simulink model "DC_core_control"  (R2023b)
settings: configuration reference "ctrl_tsk_conf" (kept outside this file)
undefined symbols (not defined in the file): ctrl_tsk_st, dcBusCtrl, shuntMaxRequestedCurrentrms
libraries: eeGeneralControl x2, simulink x1, slpidlib x1
settings Model: DataDictionary=fmuGenerationDictionay.sldd  Creator=Veimar  LastModifiedBy=Veimar
settings ConfigSetRef: SourceName=ctrl_tsk_conf

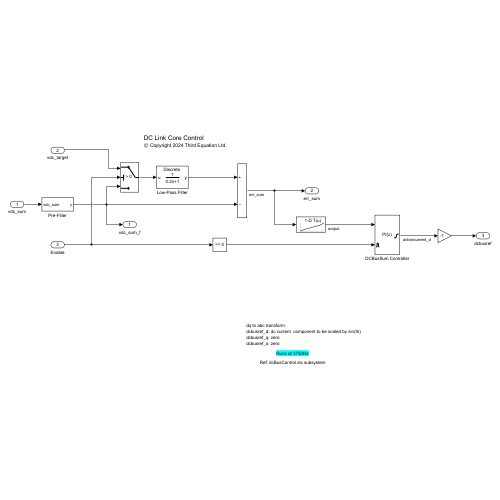
[thumbnail: Simulink's stored preview of the top-level diagram]
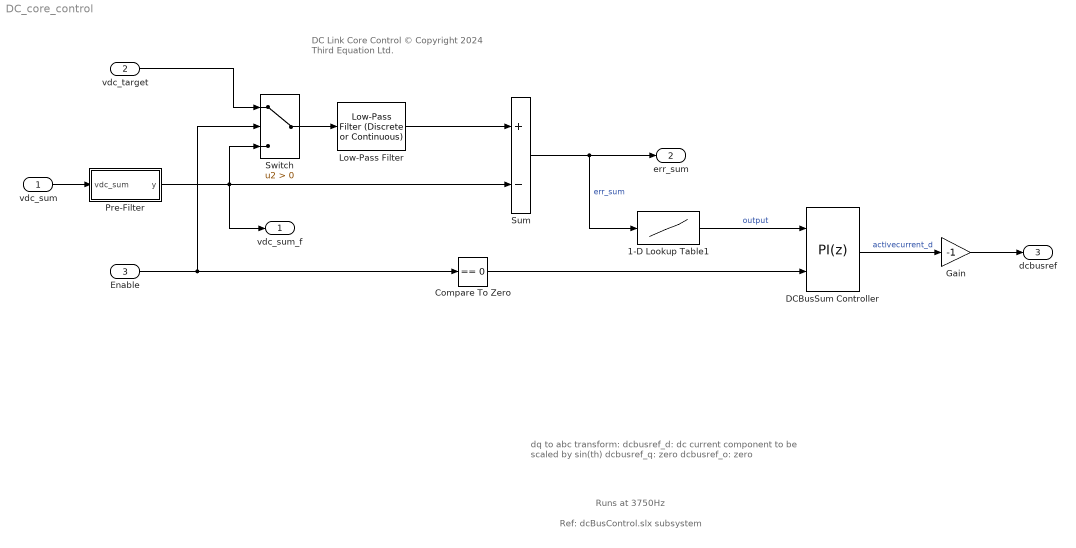
== system DC_core_control ==
  note: Runs at 3750Hz
  note: Ref: dcBusControl.slx subsystem
  note: dq to abc transform:
      | dcbusref_d: dc current  component to be scaled by sin(th)
      | dcbusref_q: zero
      | dcbusref_o: zero
  note: DC Link Core Control
      | © Copyright 2024 Third Equation Ltd.
  vdc_sum : Inport  OutDataTypeStr=single  PortDimensions=1
  vdc_target : Inport  Port=2  OutDataTypeStr=single  PortDimensions=1
  Enable : Inport  Port=3  OutDataTypeStr=boolean  PortDimensions=1
  1-D Lookup Table1 : Lookup_n-D  NumberOfTableDimensions=1  BreakpointsForDimension1=[-15 -10 10 15]  Table=[-20 -10 10 20]  InternalRulePriority=Speed  RndMeth=Simplest
  Compare To Zero : simulink/Logic and Bit Operations/Compare To Zero  relop===  OutDataTypeStr=boolean
  DCBusSum Controller : slpidlib/PID Controller  Controller=PI  Form=Parallel  TimeDomain=Discrete-time  UseExternalTs=off  SampleTime=-1  IntegratorMethod=Forward Euler  FilterMethod=Forward Euler  ControllerParametersSource=internal  P=dcBusCtrl.Sum.PGain  I=dcBusCtrl.Sum.IGain  UseKiTs=off  D=0  N=100  UseFilter=on  TunerSelectOption=Frequency Response Based  InitialConditionSource=internal  InitialConditionForIntegrator=0  InitialConditionForFilter=0  DifferentiatorICPrevScaledInput=0  ExternalReset=level  TrackingMode=off  Kt=1  LimitOutput=on  SatLimitsSource=internal  UpperSaturationLimit=shuntMaxRequestedCurrentrms*sqrt(2)  LowerSaturationLimit=-shuntMaxRequestedCurrentrms*sqrt(2)  LinearizeAsGain=on  AntiWindupMode=clamping  Kb=1  LimitIntegrator=off  UpperIntegratorSaturationLimit=inf  LowerIntegratorSaturationLimit=-inf  POutMin=[]  POutMax=[]  IOutMin=[]  IOutMax=[]  DOutMin=[]  DOutMax=[]  NOutMin=[]  NOutMax=[]  SumOutMin=[]  SumOutMax=[]  SaturationOutMin=[]  SaturationOutMax=[]  PParamMin=[]  PParamMax=[]  IParamMin=[]  IParamMax=[]  DParamMin=[]  DParamMax=[]  NParamMin=[]  NParamMax=[]  KbParamMin=[]  KbParamMax=[]  KtParamMin=[]  KtParamMax=[]  KbOutMin=[]  KbOutMax=[]  KtOutMin=[]  KtOutMax=[]  IntegratorOutMin=[]  IntegratorOutMax=[]  FilterOutMin=[]  FilterOutMax=[]  SumI1OutMin=[]  SumI1OutMax=[]  SumI2OutMin=[]  SumI2OutMax=[]  SumI3OutMin=[]  SumI3OutMax=[]  SumI4OutMin=[]  SumI4OutMax=[]  SumDOutMin=[]  SumDOutMax=[]  DifferentiatorOutMin=[]  DifferentiatorOutMax=[]  FilterDiffOutCoefMin=[]  FilterDiffOutCoefMax=[]  ReciprocalOutMin=[]  ReciprocalOutMax=[]  SumDenOutMin=[]  SumDenOutMax=[]  SumNumOutMin=[]  SumNumOutMax=[]  DivideOutMin=[]  DivideOutMax=[]  UdiffTsProdOutMin=[]  UdiffTsProdOutMax=[]  NTsProdOutMin=[]  NTsProdOutMax=[]  UintegralTsProdOutMin=[]  UintegralTsProdOutMax=[]  UngainTsProdOutMin=[]  UngainTsProdOutMax=[]  ClampingZeroOutDataTypeStr=Inherit: Inherit via back propagation  ClampingZeroOutMin=[]  ClampingZeroOutMax=[]  FilterDenConstantOutDataTypeStr=Inherit: Inherit via back propagation  FilterDenConstantOutMin=[]  FilterDenConstantOutMax=[]  PCopyOutDataTypeStr=Inherit: Inherit via back propagation  PCopyOutMin=[]  PCopyOutMax=[]  NCopyOutDataTypeStr=Inherit: Inherit via back propagation  NCopyOutMin=[]  NCopyOutMax=[]  IntegratorContinuousStateAttributes=''  IntegratorStateMustResolveToSignalObject=off  IntegratorRTWStateStorageClass=Auto  FilterContinuousStateAttributes=''  FilterStateMustResolveToSignalObject=off  FilterRTWStateStorageClass=Auto  ParallelPVariant=InternalParameters  IdealPVariant=Disabled  IVariant=InternalParameters  DVariant=Disabled  IntegratorVariant=Discrete  SatVariant=Enabled  AWVariant=DiscClampingParallel  PCopyVariant=Disabled  TRVariant=Disabled  FdbkBlocksVariant=Forward  IdealPFdbkVariant=Disabled  SatFdbkVariant=Disabled  DerivativeFilterVariant=Disabled  NVariant=Disabled  NCopyVariant=Disabled_SignalSpec  FilterICVariant=Disabled  IntegratorICVariant=InternalICs  ExternalResetVariant=ExternalReset  TRSumVariant=Passthrough  SumFdbkVariant=Disabled  SumVariant=Sum_PI  TsampFilterVariant=InternalTs  TsampNgainVariant=Passthrough  TsampIntegralVariant=Disabled_SignalSpec  ExternalSaturationOutDataTypeStr=Inherit: Same as second input
  Gain : Gain  Gain=-1
  Low-Pass Filter : eeGeneralControl/Low-Pass Filter (Discrete or Continuous)  K=1  T=0.2  B=inf  A=-inf  init_option=Inherited from block input  x0=0  Ts=-1
  Pre-Filter : Subsystem
  Sum : Sum  Inputs=+-
  Switch : Switch  Criteria=u2 > Threshold  SaturateOnIntegerOverflow=off  InputSameDT=off
  vdc_sum_f : Outport  OutDataTypeStr=single  PortDimensions=1
  err_sum : Outport  Port=2  OutDataTypeStr=single  PortDimensions=1
  dcbusref : Outport  Port=3  OutDataTypeStr=single  PortDimensions=1
  wires:
  Enable/1 -> Switch/2, Compare To Zero/1
  Sum/1 -> 1-D Lookup Table1/1, err_sum/1  "err_sum"
  Pre-Filter/1(y) -> vdc_sum_f/1, Sum/2, Switch/3
  1-D Lookup Table1/1 -> DCBusSum Controller/1  "output"
  DCBusSum Controller/1 -> Gain/1  "activecurrent_d"
  vdc_sum/1 -> Pre-Filter/1(vdc_sum)
  Gain/1 -> dcbusref/1
  Switch/1 -> Low-Pass Filter/1
  vdc_target/1 -> Switch/1
  Low-Pass Filter/1 -> Sum/1
  Compare To Zero/1 -> DCBusSum Controller/2

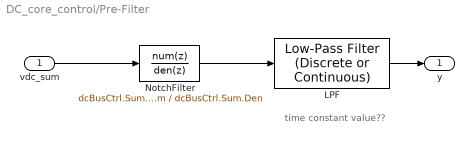
== system DC_core_control/Pre-Filter ==
  note: time constant value??
  vdc_sum : Inport
  LPF : eeGeneralControl/Low-Pass Filter (Discrete or Continuous)  K=1  T=1/(100 * 2 * pi)  B=inf  A=-inf  init_option=Inherited from block input  x0=0  Ts=ctrl_tsk_st
  NotchFilter : DiscreteFilter  Numerator=dcBusCtrl.Sum.Num  Denominator=dcBusCtrl.Sum.Den
  y : Outport
  wires:
  NotchFilter/1 -> LPF/1
  vdc_sum/1 -> NotchFilter/1
  LPF/1 -> y/1
